simulink model "PitchAngleIOLoopSystem"  (R2020a)
settings: Solver=VariableStepAuto  StartTime=0.0  StopTime=10  RelTol=1e-3
settings Model: Creator=OZAN  LastModifiedBy=OZAN

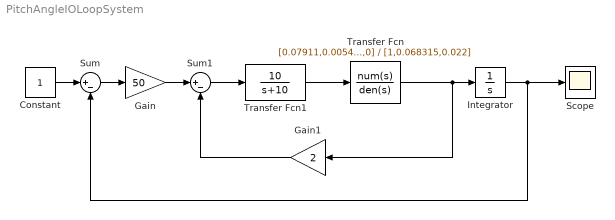
== system PitchAngleIOLoopSystem ==
  Constant : Constant
  Gain : Gain  Gain=50
  Gain1 : Gain  Gain=2
  Integrator : Integrator
  Scope : Scope
  Sum : Sum  Inputs=|+-
  Sum1 : Sum  Inputs=|+-
  Transfer Fcn : TransferFcn  Numerator=[0.07911,0.005404,0]  Denominator=[1,0.068315,0.022]
  Transfer Fcn1 : TransferFcn  Numerator=[10]  Denominator=[1 10]
  wires:
  Sum/1 -> Gain/1
  Integrator/1 -> Scope/1, Sum/2
  Gain/1 -> Sum1/1
  Sum1/1 -> Transfer Fcn1/1
  Transfer Fcn/1 -> Gain1/1, Integrator/1
  Transfer Fcn1/1 -> Transfer Fcn/1
  Gain1/1 -> Sum1/2
  Constant/1 -> Sum/1
